simulink model "RedresseurMonoPhase_DoubleAlternanceSimul"  (R2013a)
settings: Solver=FixedStepDiscrete  StartTime=0.0  StopTime=10.0  FixedStep=Tpas  RelTol=1e-3
values from neighbouring files (symbols this model uses):
  Freq = 60    [RedresseurMonoPhase_DoubleAlternance.m]    (also in RedresseurMonoPhase_SimpleAlternance.m)
  L = 0.5    [RedresseurMonoPhase_DoubleAlternance.m]    (also in RedresseurMonoPhase_SimpleAlternance.m = 0.001)
  Modulation = 1    [RedresseurMonoPhase_DoubleAlternance.m]    (also in RedresseurMonoPhase_SimpleAlternance.m = 0.5)
  PhaseDelay = 0    [RedresseurMonoPhase_DoubleAlternance.m]    (also in RedresseurMonoPhase_SimpleAlternance.m = 0.1)
  R = 2.5    [RedresseurMonoPhase_DoubleAlternance.m]    (also in RedresseurMonoPhase_SimpleAlternance.m = 1)
  Tpas = 1e-6    (= 1e-06)    [RedresseurMonoPhase_DoubleAlternance.m]    (also in RedresseurMonoPhase_SimpleAlternance.m)
  Vac = sqrt(2) * 120    [RedresseurMonoPhase_DoubleAlternance.m]    (also in RedresseurMonoPhase_SimpleAlternance.m = 1)
libraries: powerlib x13
settings Model: Creator=francisvalois  LastModifiedBy=Francis

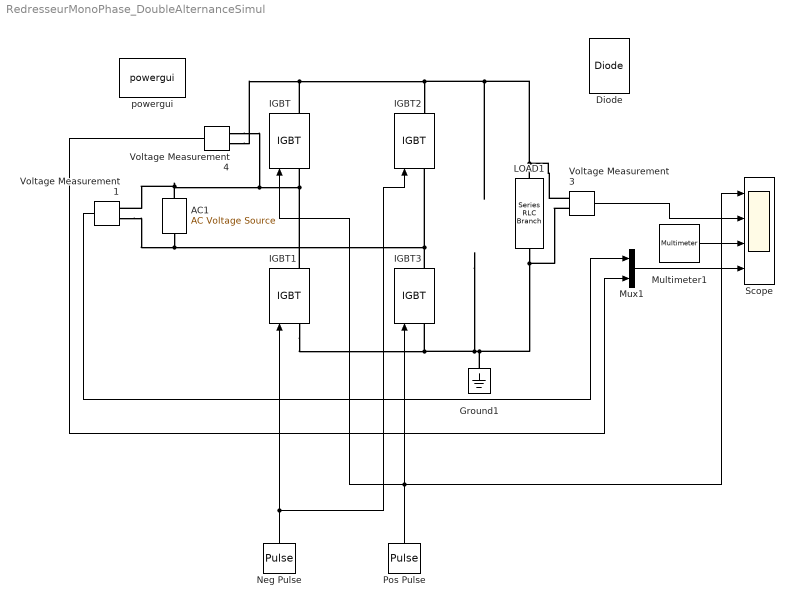
== system RedresseurMonoPhase_DoubleAlternanceSimul ==
  AC1 : powerlib/Electrical Sources/AC Voltage Source  Amplitude=Vac  Phase=0  Frequency=Freq  SampleTime=Tpas  Measurements=None
  Diode : powerlib/Power Electronics/Diode  Ron=0.001  Lon=0  Vf=0  IC=0  UseSnubber=off  Rs=500  Cs=250e-9  Measurements=on
  Ground1 : powerlib/Elements/Ground  LConnTagsString=a
  IGBT{,1..3} (4 alike) : powerlib/Power Electronics/IGBT  Ron=0.001  Lon=0  Vf=0  Tf=1e-6  Tt=2e-6  IC=0  Rs=1e5  Cs=inf  Measurements=on
  LOAD1 : powerlib/Elements/Series RLC Branch  LConnTagsString=__new0  RConnTagsString=__new0  BranchType=RL  Resistance=R  Inductance=L  SetiL0=off  InitialCurrent=0  Capacitance=1e-6  Setx0=off  InitialVoltage=0  Measurements=Branch current
  Multimeter1 : powerlib/Measurements/Multimeter  PhasorSimulation=off  OutputType=Complex  sel=1  L=1  Gain=1  yselected={'Ib: LOAD1'};  PSBOutputType=1  PSBequivalent=0  AxesSetting=[0,0.1,-100,100]  Display=0  SavedBlockNames=-11
  Mux1 : Mux  Inputs=2
  Neg Pulse : DiscretePulseGenerator  Period=floor(1/Tpas * 1/Freq)  PulseWidth=floor(1/Tpas * 1/Freq * Modulation/2)  PhaseDelay=floor(1/Tpas * 1/Freq * (1/2 + PhaseDelay/2))  SampleTime=Tpas
  Pos Pulse : DiscretePulseGenerator  Period=floor(1/Tpas * 1/Freq)  PulseWidth="floor(1/Tpas * 1/Freq * (Modulation  - PhaseDelay)/2)"  PhaseDelay=floor(1/Tpas * 1/Freq * PhaseDelay/2)  SampleTime=Tpas
  Scope : Scope  NumInputPorts=4
      settings: TimeRange=0.1666666666666667  YMin=0~-25~0~-175  YMax=1~350~60~175
  Voltage Measurement1 : powerlib/Measurements/Voltage Measurement  PhasorSimulation=off  OutputType=Complex  PSBequivalent=0
  Voltage Measurement3 : powerlib/Measurements/Voltage Measurement  PhasorSimulation=off  OutputType=Complex  PSBequivalent=0
  Voltage Measurement4 : powerlib/Measurements/Voltage Measurement  PhasorSimulation=off  OutputType=Complex  PSBequivalent=0
  powergui : powerlib/powergui  Priority=1  SimulationMode=Discrete  SolverType=Tustin  SampleTime=Tpas  frequency=60  SPID=off  DisableSnubberDevices=off  DisableRonSwitches=off  DisableVfSwitches=off  SwTol=0  Interpol=off  DisplayEquations=off  frequencyindice=60  Pbase=100e6  ErrMax=1e-4  Iterations=50  UnitsV=kV  UnitsW=MW  FunctionMessages=off  echomessages=off  HookPort=off  EnableUseOfTLC=off  x0status=blocks  RestoreLinks=warning  ResistiveCurrentMeasurement=off  Frange=[0:2:500]  Ylog=off  Xlog=on  ShowGrid=off  save=off  variable=ZData  ZoomFFT=off  StartTime=0.0  cycles=1  DisplayStyle=1  fundamental=60  FreqAxis=off  MaxFrequency=1000  frequencyindicesteady=1  RmsSteady=1  display=off  Ts=0  methode=off
  wires:
  Mux1/1 -> Scope/4
  Multimeter1/1 -> Scope/3
  Voltage Measurement3/1 -> Scope/2
  Voltage Measurement4/1 -> Mux1/2
  Voltage Measurement1/1 -> Mux1/1
  Neg Pulse/1 -> IGBT2/1, IGBT1/1
  Pos Pulse/1 -> Scope/1, IGBT/1, IGBT3/1
  connections:
  IGBT1/RConn1 -- Voltage Measurement4/LConn1 -- Voltage Measurement1/LConn1 -- AC1/RConn1 -- IGBT/LConn1
  IGBT3/RConn1 -- Voltage Measurement1/LConn2 -- AC1/LConn1 -- IGBT2/LConn1
  IGBT/RConn1 -- Voltage Measurement4/LConn2 -- Voltage Measurement3/LConn1 -- LOAD1/LConn1 -- IGBT2/RConn1
  LOAD1/RConn1 -- Ground1/LConn1 -- IGBT3/LConn1 -- IGBT1/LConn1 -- Voltage Measurement3/LConn2
